simulink model "sldemo_tc"  (R2024a)
settings: Solver=ode3  StartTime=0.0  StopTime=10.0  FixedStep=0.005  RelTol=1e-3
StartFcn:
  | set_param('sldemo_tc/Scope','Open','on')
model workspace (MAT data in the model file):
  TypeS_E_Volts = [-0.000236 -0.000232 -0.000228 -0.000224 -0.000219 -0.000215 -0.000211 -0.000207 -0.000203 -0.000199 -0.000194 -0.00019 ... (1816 elements, 1816x1)]
  TypeS_T_degC = [-50 -49 -48 -47 -46 -45 -44 -43 -42 -41 -40 -39 ... (1816 elements, 1816x1)]
  TypeS_bits_bp = [0 50 100 150 200 250 300 350 400 450 500 550 ... (83 elements, 83x1)]
  TypeS_tdegc_interp = [-50 -1.05395507812 38.4789352417 73.4326858521 105.529296875 135.797668457 164.757202148 192.63710022 219.712234497 246.231826782 272.095336914 297.6043396 ... (83 elements, 83x1)]
  TypeS_tdegc_vs_bits = [-50 -48.8466186523 -47.6932373047 -46.6318855286 -45.6364746094 -44.4830932617 -43.3297119141 -42.1763305664 -41.0229492188 -40.0956535339 -38.9661865234 -37.8502426147 ... (4096 elements, 4096x1)]
  e_vs_counts = [-0.236 -0.231386474609 -0.226772949219 -0.222159423828 -0.217545898437 -0.212932373047 -0.208318847656 -0.203705322266 -0.199091796875 -0.194478271484 -0.189864746094 -0.185251220703 ... (4096 elements, 4096x1)]
(part 2 of 2)

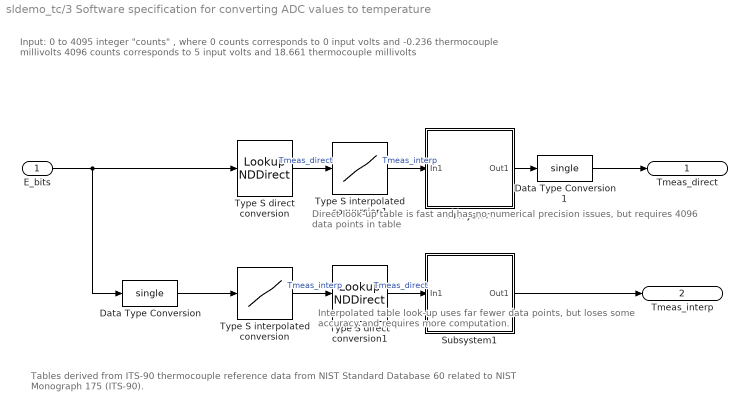
== system sldemo_tc/3 Software specification for converting ADC values to temperature ==
  note: Input: 0 to 4095 integer "counts" , where
      |             0        counts corresponds to 0 input volts and -0.236 thermocouple millivolts
      |             4096 counts corresponds to 5 input volts and 18.661 thermocouple millivolts
  note: Tables derived from ITS-90 thermocouple reference data
      | from NIST Standard Database 60 related to NIST Monograph 175 (ITS-90).
  note: Direct look-up table is fast and has no numerical precision issues,
      | but requires 4096 data points in table
  note: Interpolated table look-up uses far fewer data points,
      | but loses some accuracy and requires more computation.
  E_bits : Inport  OutDataTypeStr=uint16  Unit=count
  Data Type Conversion : DataTypeConversion  OutDataTypeStr=single  SaturateOnIntegerOverflow=off  RndMeth=Floor
  Data Type Conversion1 : DataTypeConversion  OutDataTypeStr=single  SaturateOnIntegerOverflow=off  RndMeth=Floor
  Subsystem : Subsystem
  Subsystem1 : Subsystem
  Type S direct conversion : LookupNDDirect  NumberOfTableDimensions=1  Table=TypeS_tdegc_vs_bits
      settings: AttributesFormatString=(%<mxTable>)
  Type S direct conversion1 : LookupNDDirect  NumberOfTableDimensions=1  Table=TypeS_tdegc_vs_bits
      settings: AttributesFormatString=(%<mxTable>)
  Type S interpolated conversion : Lookup_n-D  NumberOfTableDimensions=1  BreakpointsForDimension1=TypeS_bits_bp  IndexSearchMethod=Linear search  BeginIndexSearchUsingPreviousIndexResult=on  Table=TypeS_tdegc_interp  ExtrapMethod=Clip  DiagnosticForOutOfRangeInput=Warning  InternalRulePriority=Speed  RndMeth=Simplest
      settings: AttributesFormatString=(%<tableData>)
  Type S interpolated conversion1 : Lookup_n-D  NumberOfTableDimensions=1  BreakpointsForDimension1=TypeS_bits_bp  IndexSearchMethod=Linear search  BeginIndexSearchUsingPreviousIndexResult=on  Table=TypeS_tdegc_interp  ExtrapMethod=Clip  DiagnosticForOutOfRangeInput=Warning  InternalRulePriority=Speed  RndMeth=Simplest
      settings: AttributesFormatString=(%<tableData>)
  Tmeas_direct : Outport  Unit=degC  VectorParamsAs1DForOutWhenUnconnected=off
  Tmeas_interp : Outport  Port=2  Unit=degC  VectorParamsAs1DForOutWhenUnconnected=off
  wires:
  E_bits/1 -> Type S direct conversion/1, Data Type Conversion/1
  Type S direct conversion/1 -> Type S interpolated conversion1/1  "Tmeas_direct"
  Data Type Conversion/1 -> Type S interpolated conversion/1
  Type S interpolated conversion/1 -> Type S direct conversion1/1  "Tmeas_interp"
  Subsystem/1(Out1) -> Data Type Conversion1/1
  Subsystem1/1(Out1) -> Tmeas_interp/1
  Type S direct conversion1/1 -> Subsystem1/1(In1)  "Tmeas_direct"
  Type S interpolated conversion1/1 -> Subsystem/1(In1)  "Tmeas_interp"
  Data Type Conversion1/1 -> Tmeas_direct/1

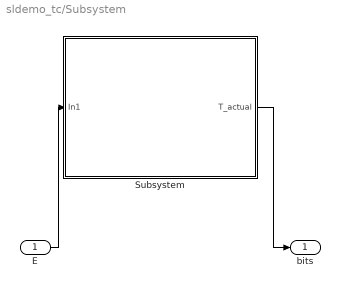
== system sldemo_tc/Subsystem ==
  E : Inport
  Subsystem : Subsystem
  bits : Outport
  wires:
  E/1 -> Subsystem/1(In1)
  Subsystem/1(T_actual) -> bits/1

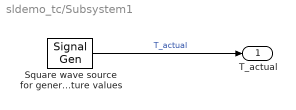
== system sldemo_tc/Subsystem1 ==
  Square wave source for generating temperature values : SignalGenerator  WaveForm=square  Amplitude=100
  T_actual : Outport
  wires:
  Square wave source for generating temperature values/1 -> T_actual/1  "T_actual"

== system sldemo_tc/z: jump to prebuilt models ==
  note: This block intentionally has no contents.

== system sldemo_tc/z: jump to table data file ==
  note: This block intentionally has no contents.

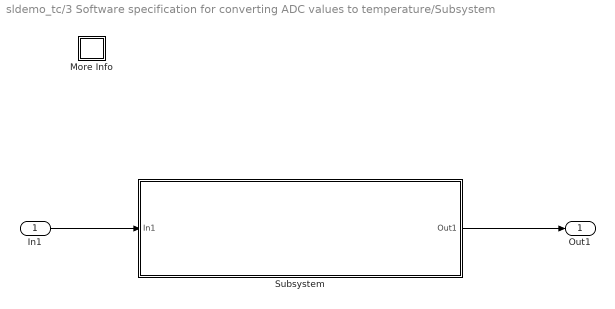
== system sldemo_tc/3 Software specification for converting ADC values to temperature/Subsystem ==
  In1 : Inport
  More Info : Subsystem
      settings: OpenFcn=showExample('simulink_general/sldemo_tc_scriptExample')
      mask Display: disp('?')
  Subsystem : Subsystem
  Out1 : Outport
  wires:
  In1/1 -> Subsystem/1(In1)
  Subsystem/1(Out1) -> Out1/1

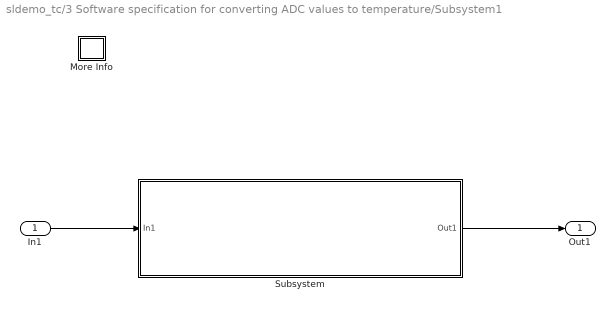
== system sldemo_tc/3 Software specification for converting ADC values to temperature/Subsystem1 ==
  In1 : Inport
  More Info : Subsystem
      settings: OpenFcn=showExample('simulink_general/sldemo_tc_scriptExample')
      mask Display: disp('?')
  Subsystem : Subsystem
  Out1 : Outport
  wires:
  Subsystem/1(Out1) -> Out1/1
  In1/1 -> Subsystem/1(In1)

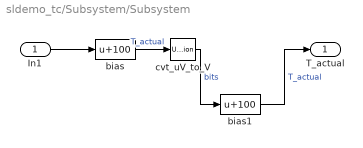
== system sldemo_tc/Subsystem/Subsystem ==
  In1 : Inport
  bias : Bias  Bias=100  SaturateOnIntegerOverflow=off
  bias1 : Bias  Bias=100  SaturateOnIntegerOverflow=off
  cvt_uV_to_V : UnitConversion
  T_actual : Outport
  wires:
  cvt_uV_to_V/1 -> bias1/1  "bits"
  bias/1 -> cvt_uV_to_V/1  "T_actual"
  In1/1 -> bias/1
  bias1/1 -> T_actual/1  "T_actual"

== system sldemo_tc/3 Software specification for converting ADC values to temperature/Subsystem/More Info ==

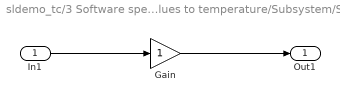
== system sldemo_tc/3 Software specification for converting ADC values to temperature/Subsystem/Subsystem ==
  In1 : Inport
  Gain : Gain
  Out1 : Outport
  wires:
  Gain/1 -> Out1/1
  In1/1 -> Gain/1

== system sldemo_tc/3 Software specification for converting ADC values to temperature/Subsystem1/More Info ==

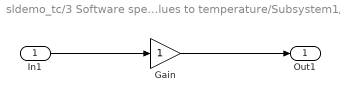
== system sldemo_tc/3 Software specification for converting ADC values to temperature/Subsystem1/Subsystem ==
  In1 : Inport
  Gain : Gain
  Out1 : Outport
  wires:
  In1/1 -> Gain/1
  Gain/1 -> Out1/1
